simulink model "AC"  (R2024b)
settings: Solver=VariableStepAuto  StartTime=0.0  StopTime=inf  RelTol=1e-3
settings Model: Creator=Umesh Reddy K  LastModifiedBy=Umesh Reddy K

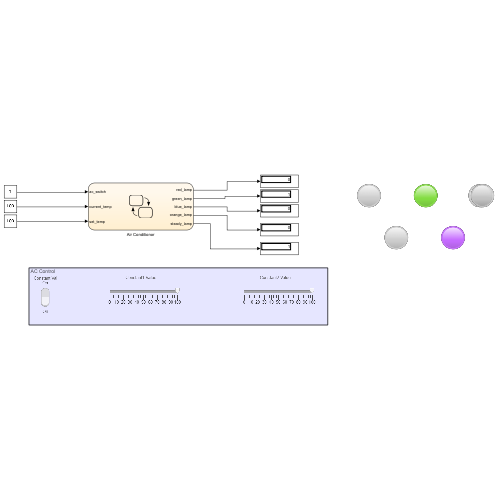
[thumbnail: Simulink's stored preview of the top-level diagram]
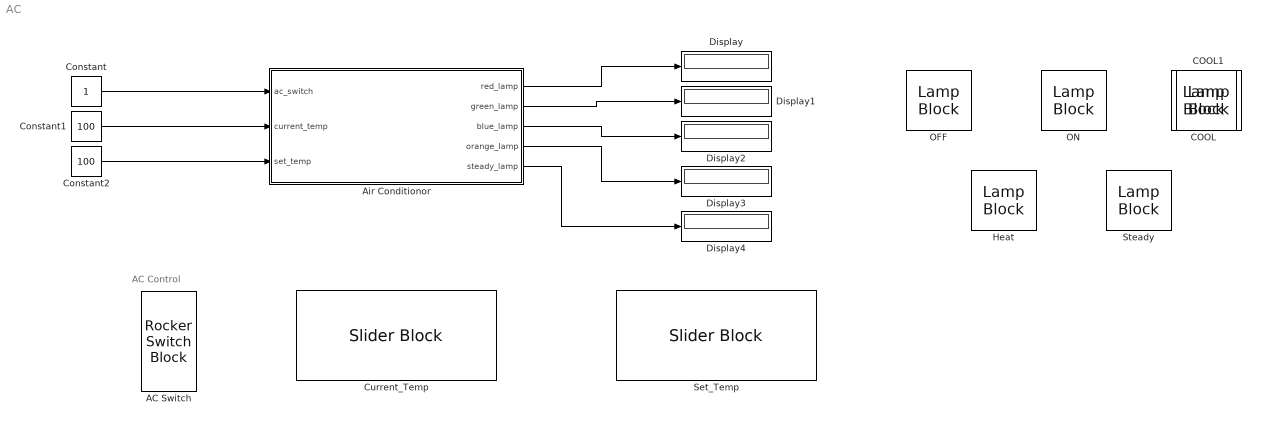
== system AC ==
  note: AC Control
  AC Switch : RockerSwitchBlock
      settings: Values={{'Off', 'On'}, [0 1]}
  Air Conditionor : Stateflow chart  TreatAsAtomicUnit=on
  COOL : LampBlock  LabelPosition=Hide
  COOL1 : LampBlock  LabelPosition=Hide
  Constant : Constant
  Constant1 : Constant  Value=100
  Constant2 : Constant  Value=100
  Current_Temp : SliderBlock
  Display{,1..4} (5 alike) : Display
  Heat : LampBlock  LabelPosition=Hide
  OFF : LampBlock  LabelPosition=Hide
  ON : LampBlock  LabelPosition=Hide
  "Set_Temp " : SliderBlock
  Steady : LampBlock  LabelPosition=Hide
  wires:
  Constant/1 -> Air Conditionor/1(ac_switch)
  Constant1/1 -> Air Conditionor/2(current_temp)
  Constant2/1 -> Air Conditionor/3(set_temp)
  Air Conditionor/1(red_lamp) -> Display/1
  Air Conditionor/2(green_lamp) -> Display1/1
  Air Conditionor/3(blue_lamp) -> Display2/1
  Air Conditionor/4(orange_lamp) -> Display3/1
  Air Conditionor/5(steady_lamp) -> Display4/1

== stateflow chart AC/Air Conditionor ==
  state COOL
    entry:
    blue_lamp = 1;
    orange_lamp = 0;
    steady_lamp = 0;
  state OFF
    entry:
    red_lamp = 1;
    green_lamp = 0;
    blue_lamp = 0;
    orange_lamp = 0;
    steady_lamp = 0;
  state ON
    entry:
    red_lamp = 0;
    green_lamp = 1;
  state HEAT
    entry:
    blue_lamp = 0;
    orange_lamp = 1;
    steady_lamp = 0;
  state STEADY
    entry:
    steady_lamp = 1;
    blue_lamp = 0;
    orange_lamp = 0;
  COOL -> STEADY [order 1] : [current_temp == set_temp]
  ON -> COOL [order 1] : [current_temp > set_temp]
  STEADY -> COOL [order 1] : [current_temp > set_temp]
  HEAT -> COOL [order 2] : [current_temp > set_temp]
  COOL -> HEAT [order 2] : [current_temp < set_temp]
  (default) -> OFF
  OFF -> ON : [ac_switch == 1]
  ON -> HEAT [order 2] : [current_temp < set_temp]
  ON -> OFF [order 3] : [ac_switch == 0]
  ON -> STEADY [order 4] : [current_temp == set_temp]
  STEADY -> HEAT [order 2] : [current_temp < set_temp]
  HEAT -> STEADY [order 1] : [current_temp == set_temp]
  data: ac_switch input; current_temp input; set_temp input; red_lamp output; green_lamp output; blue_lamp output; orange_lamp output; steady_lamp output
